simulink model "task_1_schem"  (R2024a)
settings: Solver=VariableStepAuto  StartTime=0.0  StopTime=10.0  RelTol=1e-3
undefined symbols (not defined in the file): A, a01, a02, B, C, K, k1, k2, T, T1, xi
settings Model: Creator=user  LastModifiedBy=user

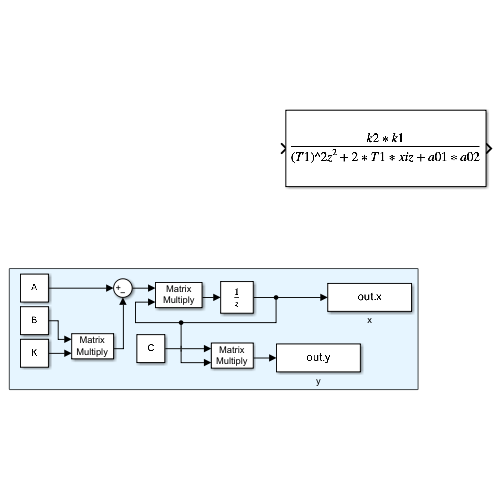
[thumbnail: Simulink's stored preview of the top-level diagram]
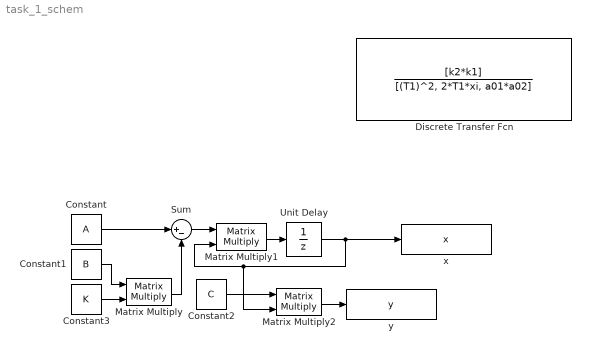
== system task_1_schem ==
  Constant : Constant  Value=A  VectorParams1D=off
  Constant1 : Constant  Value=B  VectorParams1D=off
  Constant2 : Constant  Value=C  VectorParams1D=off
  Constant3 : Constant  Value=K  VectorParams1D=off
  Discrete Transfer Fcn : DiscreteTransferFcn  Numerator=[k2*k1]  Denominator=[(T1)^2, 2*T1*xi, a01*a02]
  Matrix Multiply : Product  Multiplication=Matrix(*)
  Matrix Multiply1 : Product  Multiplication=Matrix(*)
  Matrix Multiply2 : Product  Multiplication=Matrix(*)
  Sum : Sum  Inputs=|+-
  Unit Delay : UnitDelay  InitialCondition=[1;1]  SampleTime=T  HasFrameUpgradeWarning=on
  x : ToWorkspace  VariableName=x  SaveFormat=Timeseries  SampleTime=-1
  y : ToWorkspace  VariableName=y  SaveFormat=Timeseries  SampleTime=-1
  wires:
  Constant/1 -> Sum/1
  Matrix Multiply/1 -> Sum/2
  Sum/1 -> Matrix Multiply1/1
  Matrix Multiply1/1 -> Unit Delay/1
  Constant2/1 -> Matrix Multiply2/1
  Matrix Multiply2/1 -> y/1
  Unit Delay/1 -> x/1, Matrix Multiply1/2, Matrix Multiply2/2
  Constant1/1 -> Matrix Multiply/1
  Constant3/1 -> Matrix Multiply/2
